simulink library "mylib"  (R2020a)
settings: Solver=VariableStepAuto  StartTime=0.0  StopTime=10.0  RelTol=1e-3
undefined symbols (not defined in the file): d_du_max_pu, dir_to_bus1, dir_to_bus_0L, dir_to_bus_2, dir_to_line1, dir_to_line_0L, dir_to_line_2, du_max_pu, du_ph_max_pu, Fi_0, Fi_T_H, Fi_T_L, Fi_T_M, I0_calc_0L, I0_comp_H, I0_comp_L, I0_comp_M, I0_max_0L, I2_max_2, I_diff1, I_diff2, I_diff3, I_diff4, I_diff5, I_diff_to, I_hight_CT1_G, I_hight_CT2_G, I_low_CT1, I_low_CT2, I_max1, I_max2, I_max3, I_max4, I_max5, I_min_sec_CT1, I_min_sec_CT2, I_unb, Iph_max_0L, Iph_max_2, jmp_in_zone, jmp_in_zone_0L, jmp_in_zone_2, K_dop, max_min1, only_K1_0L, only_K1_2, only_K2_0L, only_K2_2, only_K3_0L, only_K3_2, P_ctl_0, PQ_Fi_ctl_0, Q_ctl_0, S_set_0, set, set1, T_fast, T_I_ctl, T_off, T_on ... (+15)
libraries: $bdroot x184, powerlib_meascontrol x97
(part 4 of 14)

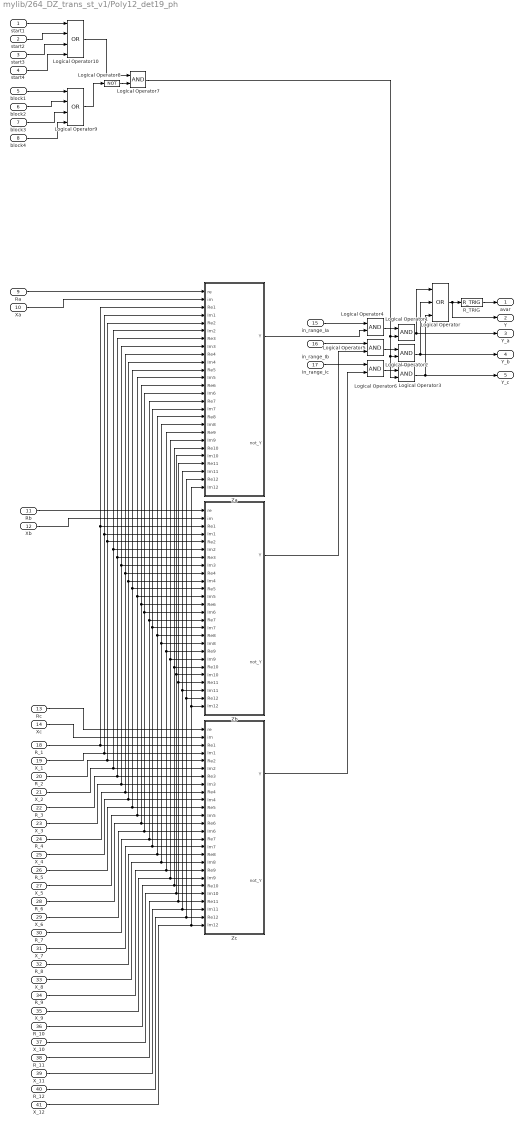
== system mylib/264_DZ_trans_st_v1/Poly12_det19_ph ==
  start1 : Inport
  start2 : Inport  Port=2
  start3 : Inport  Port=3
  start4 : Inport  Port=4
  block1 : Inport  Port=5
  block2 : Inport  Port=6
  block3 : Inport  Port=7
  block4 : Inport  Port=8
  Ra : Inport  Port=9
  Xa : Inport  Port=10
  Rb : Inport  Port=11
  Xb : Inport  Port=12
  Rc : Inport  Port=13
  Xc : Inport  Port=14
  in_range_Ia : Inport  Port=15
  in_range_Ib : Inport  Port=16
  in_range_Ic : Inport  Port=17
  R_1 : Inport  Port=18
  X_1 : Inport  Port=19
  R_2 : Inport  Port=20
  X_2 : Inport  Port=21
  R_3 : Inport  Port=22
  X_3 : Inport  Port=23
  R_4 : Inport  Port=24
  X_4 : Inport  Port=25
  R_5 : Inport  Port=26
  X_5 : Inport  Port=27
  R_6 : Inport  Port=28
  X_6 : Inport  Port=29
  R_7 : Inport  Port=30
  X_7 : Inport  Port=31
  R_8 : Inport  Port=32
  X_8 : Inport  Port=33
  R_9 : Inport  Port=34
  X_9 : Inport  Port=35
  R_10 : Inport  Port=36
  X_10 : Inport  Port=37
  R_11 : Inport  Port=38
  X_11 : Inport  Port=39
  R_12 : Inport  Port=40
  X_12 : Inport  Port=41
  Logical Operator : Logic  Operator=OR  Inputs=3  AllPortsSameDT=off  OutDataTypeStr=boolean
  Logical Operator{1..7} (7 alike) : Logic  AllPortsSameDT=off  OutDataTypeStr=boolean
  Logical Operator10 : Logic  Operator=OR  Inputs=4  AllPortsSameDT=off  OutDataTypeStr=boolean
  Logical Operator8 : Logic  Operator=NOT  AllPortsSameDT=off  OutDataTypeStr=boolean
  Logical Operator9 : Logic  Operator=OR  Inputs=4  AllPortsSameDT=off  OutDataTypeStr=boolean
  R_TRIG : $bdroot/R_TRIG  SystemSampleTime=-1  Latency=0  AutoFrameSizeCalculation=off
  Za : Subsystem
  Zb : Subsystem
  Zc : Subsystem
  avar : Outport
  Y : Outport  Port=2
  Y_a : Outport  Port=3
  Y_b : Outport  Port=4
  Y_c : Outport  Port=5
  wires:
  R_TRIG/1 -> avar/1
  Logical Operator/1 -> Y/1, R_TRIG/1
  Logical Operator1/1 -> Logical Operator/1, Y_a/1
  Logical Operator2/1 -> Logical Operator/2, Y_b/1
  Logical Operator3/1 -> Logical Operator/3, Y_c/1
  Logical Operator6/1 -> Logical Operator3/1
  Logical Operator5/1 -> Logical Operator2/1
  Logical Operator4/1 -> Logical Operator1/1
  in_range_Ia/1 -> Logical Operator4/1
  in_range_Ib/1 -> Logical Operator5/1
  in_range_Ic/1 -> Logical Operator6/1
  Logical Operator8/1 -> Logical Operator7/2
  Logical Operator7/1 -> Logical Operator3/2, Logical Operator2/2, Logical Operator1/2
  Logical Operator9/1 -> Logical Operator8/1
  Logical Operator10/1 -> Logical Operator7/1
  block1/1 -> Logical Operator9/1
  block2/1 -> Logical Operator9/2
  block3/1 -> Logical Operator9/3
  block4/1 -> Logical Operator9/4
  start4/1 -> Logical Operator10/4
  start3/1 -> Logical Operator10/3
  start2/1 -> Logical Operator10/2
  start1/1 -> Logical Operator10/1
  R_1/1 -> Za/3(Re1), Zb/3(Re1), Zc/3(Re1)
  X_1/1 -> Za/4(Im1), Zb/4(Im1), Zc/4(Im1)
  R_2/1 -> Za/5(Re2), Zb/5(Re2), Zc/5(Re2)
  X_2/1 -> Za/6(Im2), Zb/6(Im2), Zc/6(Im2)
  R_3/1 -> Za/7(Re3), Zb/7(Re3), Zc/7(Re3)
  X_3/1 -> Za/8(Im3), Zb/8(Im3), Zc/8(Im3)
  R_4/1 -> Za/9(Re4), Zb/9(Re4), Zc/9(Re4)
  X_4/1 -> Za/10(Im4), Zb/10(Im4), Zc/10(Im4)
  R_5/1 -> Za/11(Re5), Zb/11(Re5), Zc/11(Re5)
  X_5/1 -> Za/12(Im5), Zb/12(Im5), Zc/12(Im5)
  R_6/1 -> Za/13(Re6), Zb/13(Re6), Zc/13(Re6)
  X_6/1 -> Za/14(Im6), Zb/14(Im6), Zc/14(Im6)
  R_7/1 -> Za/15(Re7), Zb/15(Re7), Zc/15(Re7)
  X_7/1 -> Za/16(Im7), Zb/16(Im7), Zc/16(Im7)
  R_8/1 -> Za/17(Re8), Zb/17(Re8), Zc/17(Re8)
  X_8/1 -> Za/18(Im8), Zb/18(Im8), Zc/18(Im8)
  R_9/1 -> Za/19(Re9), Zb/19(Re9), Zc/19(Re9)
  X_9/1 -> Za/20(Im9), Zb/20(Im9), Zc/20(Im9)
  R_10/1 -> Za/21(Re10), Zb/21(Re10), Zc/21(Re10)
  X_10/1 -> Za/22(Im10), Zb/22(Im10), Zc/22(Im10)
  R_11/1 -> Za/23(Re11), Zb/23(Re11), Zc/23(Re11)
  X_11/1 -> Za/24(Im11), Zb/24(Im11), Zc/24(Im11)
  R_12/1 -> Za/25(Re12), Zb/25(Re12), Zc/25(Re12)
  X_12/1 -> Za/26(Im12), Zb/26(Im12), Zc/26(Im12)
  Xc/1 -> Zc/2(im)
  Rc/1 -> Zc/1(re)
  Rb/1 -> Zb/1(re)
  Xb/1 -> Zb/2(im)
  Xa/1 -> Za/2(im)
  Ra/1 -> Za/1(re)
  Za/1(Y) -> Logical Operator4/2
  Zb/1(Y) -> Logical Operator5/2
  Zc/1(Y) -> Logical Operator6/2

== system mylib/264_DZ_trans_st_v1/St1 ==
  fast1_time : Inport
  fast2_time : Inport  Port=2
  fast1_zero : Inport  Port=3
  fast2_zero : Inport  Port=4
  block1 : Inport  Port=5
  block2 : Inport  Port=6
  block3 : Inport  Port=7
  block4 : Inport  Port=8
  in_a : Inport  Port=9
  in_b : Inport  Port=10
  in_c : Inport  Port=11
  alt_in_a : Inport  Port=12
  alt_in_b : Inport  Port=13
  alt_in_c : Inport  Port=14
  jmp_a : Inport  Port=15
  jmp_b : Inport  Port=16
  jmp_c : Inport  Port=17
  1 : Logic  Operator=OR  Inputs=4  AllPortsSameDT=off  OutDataTypeStr=boolean
  Constant1 : Constant  Value=only_K2
  Constant2 : Constant  Value=only_K3
  Constant3 : Constant  Value=only_K1
  Constant4 : Constant  Value=jmp_in_zone
  Logical Operator1 : Logic  Operator=OR  Inputs=3  AllPortsSameDT=off  OutDataTypeStr=boolean
  Logical Operator10 : Logic  Inputs=3  AllPortsSameDT=off  OutDataTypeStr=boolean
  Logical Operator{2,4,6,11..13} (6 alike) : Logic  AllPortsSameDT=off  OutDataTypeStr=boolean
  Logical Operator{14,16..17,27..28} (5 alike) : Logic  Operator=OR  AllPortsSameDT=off  OutDataTypeStr=boolean
  Logical Operator26 : Logic  Operator=OR  Inputs=3  AllPortsSameDT=off  OutDataTypeStr=boolean
  Logical Operator3 : Logic  Operator=NOT  AllPortsSameDT=off  OutDataTypeStr=boolean
  Logical Operator5 : Logic  Operator=NOT  AllPortsSameDT=off  OutDataTypeStr=boolean
  Logical Operator7 : Logic  Operator=NOT  AllPortsSameDT=off  OutDataTypeStr=boolean
  Logical Operator8 : Logic  Inputs=3  AllPortsSameDT=off  OutDataTypeStr=boolean
  Logical Operator9 : Logic  Inputs=3  AllPortsSameDT=off  OutDataTypeStr=boolean
  R_TRIG : $bdroot/R_TRIG  SystemSampleTime=-1  Latency=0  AutoFrameSizeCalculation=off
  Subsystem : Subsystem  mask{time=[T_fast, T_st]}
      mask prompts: time "time [T_fast, T_st]"
  in_1 : Subsystem  mask{in_jmp=[T_reset]}
      mask prompts: in_jmp "in_jmp[T_reset]"
  in_2 : Subsystem  mask{in_jmp=[T_reset]}
      mask prompts: in_jmp "in_jmp[T_reset]"
  in_3 : Subsystem  mask{in_jmp=[T_reset]}
      mask prompts: in_jmp "in_jmp[T_reset]"
  k_type : Subsystem
  out_a : $bdroot/out3  out=[T_out]
  out_b : $bdroot/out3  out=[T_out]
  out_c : $bdroot/out3  out=[T_out]
  avar : Outport
  Y : Outport  Port=2
  Y_a : Outport  Port=3
  Y_b : Outport  Port=4
  Y_c : Outport  Port=5
  fast : Outport  Port=6
  fast_a : Outport  Port=7
  fast_b : Outport  Port=8
  fast_c : Outport  Port=9
  wires:
  fast1_time/1 -> Logical Operator27/1
  fast2_zero/1 -> Logical Operator28/2
  fast1_zero/1 -> Logical Operator28/1
  fast2_time/1 -> Logical Operator27/2
  block1/1 -> 1/1
  block2/1 -> 1/2
  block3/1 -> 1/3
  block4/1 -> 1/4
  in_a/1 -> in_1/2(in), Logical Operator8/1
  in_c/1 -> in_3/2(in), Logical Operator10/1
  Logical Operator26/1 -> Y/1, R_TRIG/1
  R_TRIG/1 -> avar/1
  in_b/1 -> in_2/2(in), Logical Operator9/1
  Constant4/1 -> in_3/1(jmp_in_zone), in_2/1(jmp_in_zone), in_1/1(jmp_in_zone)
  jmp_a/1 -> in_1/3(jmp)
  jmp_b/1 -> in_2/3(jmp)
  jmp_c/1 -> in_3/3(jmp)
  Logical Operator3/1 -> Logical Operator2/1
  in_1/1(Y) -> Logical Operator2/2  "Ya"
  Logical Operator5/1 -> Logical Operator4/1
  in_2/1(Y) -> Logical Operator4/2  "Yb"
  Logical Operator7/1 -> Logical Operator6/1
  in_3/1(Y) -> Logical Operator6/2  "Yc"
  1/1 -> Logical Operator7/1, Logical Operator5/1, Logical Operator3/1
  out_a/1 -> Logical Operator26/1, Y_a/1  "Y_c"
  out_b/1 -> Logical Operator26/2, Y_b/1  "Y_c"
  out_c/1 -> Logical Operator26/3, Y_c/1  "Y_c"
  Logical Operator8/1 -> out_a/1
  Logical Operator9/1 -> out_b/1
  Logical Operator10/1 -> out_c/1
  Subsystem/3(Out3) -> Logical Operator10/2
  Subsystem/2(Out2) -> Logical Operator9/2
  Subsystem/1(Out1) -> Logical Operator8/2
  Logical Operator2/1 -> Logical Operator1/1, fast_a/1, Logical Operator11/2, k_type/1(In_a)
  Logical Operator4/1 -> Logical Operator1/2, fast_b/1, Logical Operator12/2, k_type/2(In_b)
  Logical Operator6/1 -> Logical Operator1/3, fast_c/1, Logical Operator13/2, k_type/3(In_ c)
  Constant3/1 -> k_type/4(only_K1)
  Constant1/1 -> k_type/5(only_K2)
  Constant2/1 -> k_type/6(only_K3)
  k_type/1(out) -> Logical Operator10/3, Logical Operator9/3, Logical Operator8/3, Logical Operator12/1, Logical Operator13/1, Logical Operator11/1
  Logical Operator11/1 -> Logical Operator14/1
  Logical Operator12/1 -> Logical Operator16/1
  Logical Operator13/1 -> Logical Operator17/1
  Logical Operator17/1 -> Subsystem/5("In3 ")
  Logical Operator16/1 -> Subsystem/4("In2 ")
  Logical Operator14/1 -> Subsystem/3("In1 ")
  alt_in_a/1 -> Logical Operator14/2
  alt_in_b/1 -> Logical Operator16/2
  alt_in_c/1 -> Logical Operator17/2
  Logical Operator27/1 -> Subsystem/1(T_fast_time)
  Logical Operator28/1 -> Subsystem/2(T_fast_zero)
  Logical Operator1/1 -> fast/1

== system mylib/264_DZ_trans_st_v1/St2 ==
  fast1_time : Inport
  fast2_time : Inport  Port=2
  fast1_zero : Inport  Port=3
  fast2_zero : Inport  Port=4
  block1 : Inport  Port=5
  block2 : Inport  Port=6
  block3 : Inport  Port=7
  block4 : Inport  Port=8
  in_a : Inport  Port=9
  in_b : Inport  Port=10
  in_c : Inport  Port=11
  alt_in_a : Inport  Port=12
  alt_in_b : Inport  Port=13
  alt_in_c : Inport  Port=14
  jmp_a : Inport  Port=15
  jmp_b : Inport  Port=16
  jmp_c : Inport  Port=17
  1 : Logic  Operator=OR  Inputs=4  AllPortsSameDT=off  OutDataTypeStr=boolean
  Constant1 : Constant  Value=only_K2
  Constant2 : Constant  Value=only_K3
  Constant3 : Constant  Value=only_K1
  Constant4 : Constant  Value=jmp_in_zone
  Logical Operator1 : Logic  Operator=OR  Inputs=3  AllPortsSameDT=off  OutDataTypeStr=boolean
  Logical Operator10 : Logic  Inputs=3  AllPortsSameDT=off  OutDataTypeStr=boolean
  Logical Operator{2,4,6,11..13} (6 alike) : Logic  AllPortsSameDT=off  OutDataTypeStr=boolean
  Logical Operator{14,16..17,27..28} (5 alike) : Logic  Operator=OR  AllPortsSameDT=off  OutDataTypeStr=boolean
  Logical Operator26 : Logic  Operator=OR  Inputs=3  AllPortsSameDT=off  OutDataTypeStr=boolean
  Logical Operator3 : Logic  Operator=NOT  AllPortsSameDT=off  OutDataTypeStr=boolean
  Logical Operator5 : Logic  Operator=NOT  AllPortsSameDT=off  OutDataTypeStr=boolean
  Logical Operator7 : Logic  Operator=NOT  AllPortsSameDT=off  OutDataTypeStr=boolean
  Logical Operator8 : Logic  Inputs=3  AllPortsSameDT=off  OutDataTypeStr=boolean
  Logical Operator9 : Logic  Inputs=3  AllPortsSameDT=off  OutDataTypeStr=boolean
  R_TRIG : $bdroot/R_TRIG  SystemSampleTime=-1  Latency=0  AutoFrameSizeCalculation=off
  Subsystem : Subsystem  mask{time=[T_fast, T_st]}
      mask prompts: time "time [T_fast, T_st]"
  in_1 : Subsystem  mask{in_jmp=[T_reset]}
      mask prompts: in_jmp "in_jmp[T_reset]"
  in_2 : Subsystem  mask{in_jmp=[T_reset]}
      mask prompts: in_jmp "in_jmp[T_reset]"
  in_3 : Subsystem  mask{in_jmp=[T_reset]}
      mask prompts: in_jmp "in_jmp[T_reset]"
  k_type : Subsystem
  out_a : $bdroot/out3  out=[T_out]
  out_b : $bdroot/out3  out=[T_out]
  out_c : $bdroot/out3  out=[T_out]
  avar : Outport
  Y : Outport  Port=2
  Y_a : Outport  Port=3
  Y_b : Outport  Port=4
  Y_c : Outport  Port=5
  fast : Outport  Port=6
  fast_a : Outport  Port=7
  fast_b : Outport  Port=8
  fast_c : Outport  Port=9
  wires:
  fast1_time/1 -> Logical Operator27/1
  fast2_zero/1 -> Logical Operator28/2
  fast1_zero/1 -> Logical Operator28/1
  fast2_time/1 -> Logical Operator27/2
  block1/1 -> 1/1
  block2/1 -> 1/2
  block3/1 -> 1/3
  block4/1 -> 1/4
  in_a/1 -> in_1/2(in), Logical Operator8/1
  in_c/1 -> in_3/2(in), Logical Operator10/1
  Logical Operator26/1 -> Y/1, R_TRIG/1
  R_TRIG/1 -> avar/1
  in_b/1 -> in_2/2(in), Logical Operator9/1
  Constant4/1 -> in_3/1(jmp_in_zone), in_2/1(jmp_in_zone), in_1/1(jmp_in_zone)
  jmp_a/1 -> in_1/3(jmp)
  jmp_b/1 -> in_2/3(jmp)
  jmp_c/1 -> in_3/3(jmp)
  Logical Operator3/1 -> Logical Operator2/1
  in_1/1(Y) -> Logical Operator2/2  "Ya"
  Logical Operator5/1 -> Logical Operator4/1
  in_2/1(Y) -> Logical Operator4/2  "Yb"
  Logical Operator7/1 -> Logical Operator6/1
  in_3/1(Y) -> Logical Operator6/2  "Yc"
  1/1 -> Logical Operator7/1, Logical Operator5/1, Logical Operator3/1
  out_a/1 -> Logical Operator26/1, Y_a/1  "Y_c"
  out_b/1 -> Logical Operator26/2, Y_b/1  "Y_c"
  out_c/1 -> Logical Operator26/3, Y_c/1  "Y_c"
  Logical Operator8/1 -> out_a/1
  Logical Operator9/1 -> out_b/1
  Logical Operator10/1 -> out_c/1
  Subsystem/3(Out3) -> Logical Operator10/2
  Subsystem/2(Out2) -> Logical Operator9/2
  Subsystem/1(Out1) -> Logical Operator8/2
  Logical Operator2/1 -> Logical Operator1/1, fast_a/1, Logical Operator11/2, k_type/1(In_a)
  Logical Operator4/1 -> Logical Operator1/2, fast_b/1, Logical Operator12/2, k_type/2(In_b)
  Logical Operator6/1 -> Logical Operator1/3, fast_c/1, Logical Operator13/2, k_type/3(In_ c)
  Constant3/1 -> k_type/4(only_K1)
  Constant1/1 -> k_type/5(only_K2)
  Constant2/1 -> k_type/6(only_K3)
  k_type/1(out) -> Logical Operator10/3, Logical Operator9/3, Logical Operator8/3, Logical Operator12/1, Logical Operator13/1, Logical Operator11/1
  Logical Operator11/1 -> Logical Operator14/1
  Logical Operator12/1 -> Logical Operator16/1
  Logical Operator13/1 -> Logical Operator17/1
  Logical Operator17/1 -> Subsystem/5("In3 ")
  Logical Operator16/1 -> Subsystem/4("In2 ")
  Logical Operator14/1 -> Subsystem/3("In1 ")
  alt_in_a/1 -> Logical Operator14/2
  alt_in_b/1 -> Logical Operator16/2
  alt_in_c/1 -> Logical Operator17/2
  Logical Operator27/1 -> Subsystem/1(T_fast_time)
  Logical Operator28/1 -> Subsystem/2(T_fast_zero)
  Logical Operator1/1 -> fast/1

== system mylib/264_DZ_trans_st_v1/St3 ==
  fast1_time : Inport
  fast2_time : Inport  Port=2
  fast1_zero : Inport  Port=3
  fast2_zero : Inport  Port=4
  block1 : Inport  Port=5
  block2 : Inport  Port=6
  block3 : Inport  Port=7
  block4 : Inport  Port=8
  in_a : Inport  Port=9
  in_b : Inport  Port=10
  in_c : Inport  Port=11
  alt_in_a : Inport  Port=12
  alt_in_b : Inport  Port=13
  alt_in_c : Inport  Port=14
  jmp_a : Inport  Port=15
  jmp_b : Inport  Port=16
  jmp_c : Inport  Port=17
  1 : Logic  Operator=OR  Inputs=4  AllPortsSameDT=off  OutDataTypeStr=boolean
  Constant1 : Constant  Value=only_K2
  Constant2 : Constant  Value=only_K3
  Constant3 : Constant  Value=only_K1
  Constant4 : Constant  Value=jmp_in_zone
  Logical Operator1 : Logic  Operator=OR  Inputs=3  AllPortsSameDT=off  OutDataTypeStr=boolean
  Logical Operator10 : Logic  Inputs=3  AllPortsSameDT=off  OutDataTypeStr=boolean
  Logical Operator{2,4,6,11..13} (6 alike) : Logic  AllPortsSameDT=off  OutDataTypeStr=boolean
  Logical Operator{14,16..17,27..28} (5 alike) : Logic  Operator=OR  AllPortsSameDT=off  OutDataTypeStr=boolean
  Logical Operator26 : Logic  Operator=OR  Inputs=3  AllPortsSameDT=off  OutDataTypeStr=boolean
  Logical Operator3 : Logic  Operator=NOT  AllPortsSameDT=off  OutDataTypeStr=boolean
  Logical Operator5 : Logic  Operator=NOT  AllPortsSameDT=off  OutDataTypeStr=boolean
  Logical Operator7 : Logic  Operator=NOT  AllPortsSameDT=off  OutDataTypeStr=boolean
  Logical Operator8 : Logic  Inputs=3  AllPortsSameDT=off  OutDataTypeStr=boolean
  Logical Operator9 : Logic  Inputs=3  AllPortsSameDT=off  OutDataTypeStr=boolean
  R_TRIG : $bdroot/R_TRIG  SystemSampleTime=-1  Latency=0  AutoFrameSizeCalculation=off
  Subsystem : Subsystem  mask{time=[T_fast, T_st]}
      mask prompts: time "time [T_fast, T_st]"
  in_1 : Subsystem  mask{in_jmp=[T_reset]}
      mask prompts: in_jmp "in_jmp[T_reset]"
  in_2 : Subsystem  mask{in_jmp=[T_reset]}
      mask prompts: in_jmp "in_jmp[T_reset]"
  in_3 : Subsystem  mask{in_jmp=[T_reset]}
      mask prompts: in_jmp "in_jmp[T_reset]"
  k_type : Subsystem
  out_a : $bdroot/out3  out=[T_out]
  out_b : $bdroot/out3  out=[T_out]
  out_c : $bdroot/out3  out=[T_out]
  avar : Outport
  Y : Outport  Port=2
  Y_a : Outport  Port=3
  Y_b : Outport  Port=4
  Y_c : Outport  Port=5
  fast : Outport  Port=6
  fast_a : Outport  Port=7
  fast_b : Outport  Port=8
  fast_c : Outport  Port=9
  wires:
  fast1_time/1 -> Logical Operator27/1
  fast2_zero/1 -> Logical Operator28/2
  fast1_zero/1 -> Logical Operator28/1
  fast2_time/1 -> Logical Operator27/2
  block1/1 -> 1/1
  block2/1 -> 1/2
  block3/1 -> 1/3
  block4/1 -> 1/4
  in_a/1 -> in_1/2(in), Logical Operator8/1
  in_c/1 -> in_3/2(in), Logical Operator10/1
  Logical Operator26/1 -> Y/1, R_TRIG/1
  R_TRIG/1 -> avar/1
  in_b/1 -> in_2/2(in), Logical Operator9/1
  Constant4/1 -> in_3/1(jmp_in_zone), in_2/1(jmp_in_zone), in_1/1(jmp_in_zone)
  jmp_a/1 -> in_1/3(jmp)
  jmp_b/1 -> in_2/3(jmp)
  jmp_c/1 -> in_3/3(jmp)
  Logical Operator3/1 -> Logical Operator2/1
  in_1/1(Y) -> Logical Operator2/2  "Ya"
  Logical Operator5/1 -> Logical Operator4/1
  in_2/1(Y) -> Logical Operator4/2  "Yb"
  Logical Operator7/1 -> Logical Operator6/1
  in_3/1(Y) -> Logical Operator6/2  "Yc"
  1/1 -> Logical Operator7/1, Logical Operator5/1, Logical Operator3/1
  out_a/1 -> Logical Operator26/1, Y_a/1  "Y_c"
  out_b/1 -> Logical Operator26/2, Y_b/1  "Y_c"
  out_c/1 -> Logical Operator26/3, Y_c/1  "Y_c"
  Logical Operator8/1 -> out_a/1
  Logical Operator9/1 -> out_b/1
  Logical Operator10/1 -> out_c/1
  Subsystem/3(Out3) -> Logical Operator10/2
  Subsystem/2(Out2) -> Logical Operator9/2
  Subsystem/1(Out1) -> Logical Operator8/2
  Logical Operator2/1 -> Logical Operator1/1, fast_a/1, Logical Operator11/2, k_type/1(In_a)
  Logical Operator4/1 -> Logical Operator1/2, fast_b/1, Logical Operator12/2, k_type/2(In_b)
  Logical Operator6/1 -> Logical Operator1/3, fast_c/1, Logical Operator13/2, k_type/3(In_ c)
  Constant3/1 -> k_type/4(only_K1)
  Constant1/1 -> k_type/5(only_K2)
  Constant2/1 -> k_type/6(only_K3)
  k_type/1(out) -> Logical Operator10/3, Logical Operator9/3, Logical Operator8/3, Logical Operator12/1, Logical Operator13/1, Logical Operator11/1
  Logical Operator11/1 -> Logical Operator14/1
  Logical Operator12/1 -> Logical Operator16/1
  Logical Operator13/1 -> Logical Operator17/1
  Logical Operator17/1 -> Subsystem/5("In3 ")
  Logical Operator16/1 -> Subsystem/4("In2 ")
  Logical Operator14/1 -> Subsystem/3("In1 ")
  alt_in_a/1 -> Logical Operator14/2
  alt_in_b/1 -> Logical Operator16/2
  alt_in_c/1 -> Logical Operator17/2
  Logical Operator27/1 -> Subsystem/1(T_fast_time)
  Logical Operator28/1 -> Subsystem/2(T_fast_zero)
  Logical Operator1/1 -> fast/1

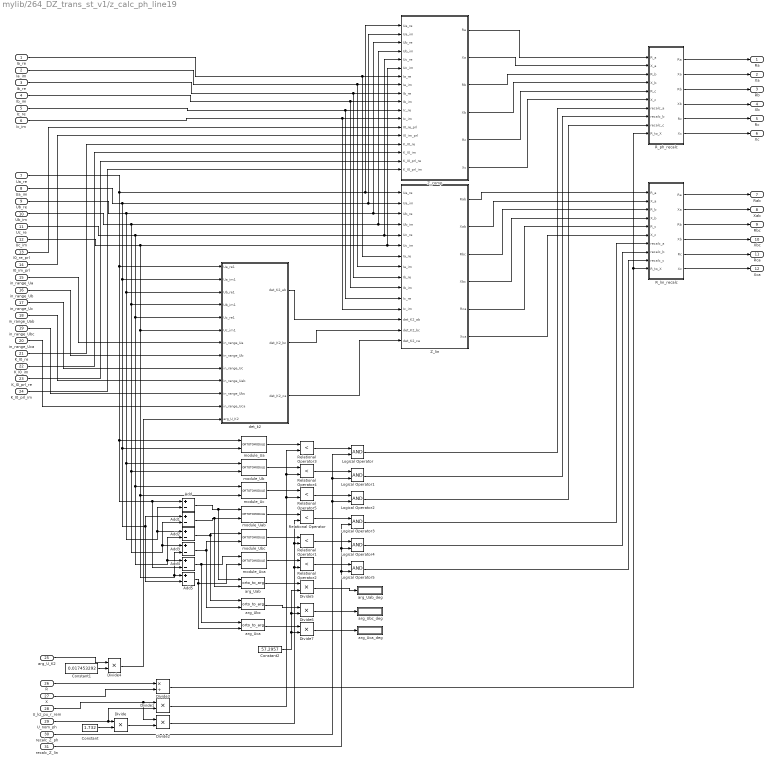
== system mylib/264_DZ_trans_st_v1/z_calc_ph_line19 ==
  Ia_re : Inport
  Ia_im : Inport  Port=2
  Ib_re : Inport  Port=3
  Ib_im : Inport  Port=4
  Ic_re : Inport  Port=5
  Ic_im : Inport  Port=6
  Ua_re : Inport  Port=7
  Ua_im : Inport  Port=8
  Ub_re : Inport  Port=9
  Ub_im : Inport  Port=10
  Uc_re : Inport  Port=11
  Uc_im : Inport  Port=12
  I0_re_prl : Inport  Port=13
  I0_im_prl : Inport  Port=14
  in_range_Ua : Inport  Port=15
  in_range_Ub : Inport  Port=16
  in_range_Uc : Inport  Port=17
  in_range_Uab : Inport  Port=18
  in_range_Ubc : Inport  Port=19
  in_range_Uca : Inport  Port=20
  K_I0_re : Inport  Port=21
  K_I0_im : Inport  Port=22
  K_I0_prl_re : Inport  Port=23
  K_I0_prl_im : Inport  Port=24
  arg_U_K2 : Inport  Port=25
  R : Inport  Port=26
  X : Inport  Port=27
  U_kz_pu_r_rem : Inport  Port=28
  U_nom_ph : Inport  Port=29
  recalc_Z_ph : Inport  Port=30
  recalc_Z_lin : Inport  Port=31
  Add{,1..5} (6 alike) : Sum  Inputs=+-
  Constant : Constant  Value=1.732
  Constant1 : Constant  Value=0.017453292
  Constant2 : Constant  Value=57.2957
  Divide{,1..2,4..7} (7 alike) : Product  Inputs=**
  Divide3 : Product  Inputs=*/
  Logical Operator{,1..5} (6 alike) : Logic  AllPortsSameDT=off  OutDataTypeStr=boolean
  R_lin_recalc : Subsystem
  R_ph_recalc : Subsystem
  Relational Operator{,1..5} (6 alike) : RelationalOperator  Operator=<  OutDataTypeStr=boolean  RndMeth=Simplest
  Z_comp : Subsystem
  Z_lin : Subsystem
  arg_Uab : $bdroot/orto_to_arg  SystemSampleTime=-1  Latency=0  AutoFrameSizeCalculation=off
  arg_Uab_deg : Display
  arg_Ubc : $bdroot/orto_to_arg  SystemSampleTime=-1  Latency=0  AutoFrameSizeCalculation=off
  arg_Ubc_deg : Display
  arg_Uca : $bdroot/orto_to_arg  SystemSampleTime=-1  Latency=0  AutoFrameSizeCalculation=off
  arg_Uca_deg : Display
  det_k2 : Subsystem
  module_Ua : $bdroot/ORTOTOMODULE  SystemSampleTime=-1  Latency=0  AutoFrameSizeCalculation=off
  module_Uab : $bdroot/ORTOTOMODULE  SystemSampleTime=-1  Latency=0  AutoFrameSizeCalculation=off
  module_Ub : $bdroot/ORTOTOMODULE  SystemSampleTime=-1  Latency=0  AutoFrameSizeCalculation=off
  module_Ubc : $bdroot/ORTOTOMODULE  SystemSampleTime=-1  Latency=0  AutoFrameSizeCalculation=off
  module_Uc : $bdroot/ORTOTOMODULE  SystemSampleTime=-1  Latency=0  AutoFrameSizeCalculation=off
  module_Uca : $bdroot/ORTOTOMODULE  SystemSampleTime=-1  Latency=0  AutoFrameSizeCalculation=off
  Ra : Outport
  Xa : Outport  Port=2
  Rb : Outport  Port=3
  Xb : Outport  Port=4
  Rc : Outport  Port=5
  Xc : Outport  Port=6
  Rab : Outport  Port=7
  Xab : Outport  Port=8
  Rbc : Outport  Port=9
  Xbc : Outport  Port=10
  Rca : Outport  Port=11
  Xca : Outport  Port=12
  wires:
  Ua_re/1 -> Z_lin/1(Ua_re), Z_comp/1(Ua_re), module_Ua/1, Add4/2, Add/1, det_k2/1(Ua_re1)
  Ub_re/1 -> det_k2/3(Ub_re1), Add/2, Add2/1, module_Ub/1, Z_comp/3(Ub_re), Z_lin/3(Ub_re)
  Ua_im/1 -> det_k2/2(Ua_im1), Add1/1, Add5/2, module_Ua/2, Z_comp/2(Ua_im), Z_lin/2(Ua_im)
  Ub_im/1 -> det_k2/4(Ub_im1), Add1/2, Add3/1, module_Ub/2, Z_comp/4(Ub_im), Z_lin/4(Ub_im)
  Uc_re/1 -> det_k2/5(Uc_re1), Add2/2, Add4/1, module_Uc/1, Z_comp/5(Uc_re), Z_lin/5(Uc_re)
  Uc_im/1 -> det_k2/6(Uc_im1), Add3/2, Add5/1, module_Uc/2, Z_comp/6(Uc_im), Z_lin/6(Uc_im)
  Add1/1 -> arg_Uab/2, module_Uab/2
  Add/1 -> module_Uab/1, arg_Uab/1
  Add2/1 -> arg_Ubc/1, module_Ubc/1
  Add3/1 -> arg_Ubc/2, module_Ubc/2
  Add4/1 -> arg_Uca/1, module_Uca/1
  Add5/1 -> arg_Uca/2, module_Uca/2
  module_Uab/1 -> Relational Operator/1
  module_Uca/1 -> Relational Operator2/1
  module_Ubc/1 -> Relational Operator1/1
  Constant/1 -> Divide/2
  U_kz_pu_r_rem/1 -> Divide2/1, Divide1/1
  U_nom_ph/1 -> Divide1/2, Divide/1
  Divide/1 -> Divide2/2
  X/1 -> Divide3/2
  R/1 -> Divide3/1
  arg_U_K2/1 -> Divide4/1
  Constant1/1 -> Divide4/2
  module_Ua/1 -> Relational Operator3/1
  module_Ub/1 -> Relational Operator4/1
  module_Uc/1 -> Relational Operator5/1
  Relational Operator3/1 -> Logical Operator/1
  Relational Operator4/1 -> Logical Operator1/1
  Relational Operator5/1 -> Logical Operator2/1
  Relational Operator/1 -> Logical Operator3/1
  Relational Operator1/1 -> Logical Operator4/1
  Relational Operator2/1 -> Logical Operator5/1
  recalc_Z_ph/1 -> Logical Operator2/2, Logical Operator1/2, Logical Operator/2
  recalc_Z_lin/1 -> Logical Operator5/2, Logical Operator4/2, Logical Operator3/2
  arg_Uab/1 -> Divide5/1
  arg_Ubc/1 -> Divide6/1
  arg_Uca/1 -> Divide7/1
  Constant2/1 -> Divide5/2, Divide6/2, Divide7/2
  Divide5/1 -> arg_Uab_deg/1
  Divide6/1 -> arg_Ubc_deg/1
  Divide7/1 -> arg_Uca_deg/1
  Divide1/1 -> Relational Operator5/2, Relational Operator3/2, Relational Operator4/2
  Divide2/1 -> Relational Operator2/2, Relational Operator1/2, Relational Operator/2
  R_ph_recalc/1(Ra) -> Ra/1
  R_ph_recalc/6(Xc) -> Xc/1
  R_ph_recalc/5(Rc) -> Rc/1
  R_ph_recalc/4(Xb) -> Xb/1
  R_ph_recalc/3(Rb) -> Rb/1
  R_ph_recalc/2(Xa) -> Xa/1
  R_lin_recalc/1(Ra) -> Rab/1
  R_lin_recalc/6(Xc) -> Xca/1
  R_lin_recalc/5(Rc) -> Rca/1
  R_lin_recalc/4(Xb) -> Xbc/1
  R_lin_recalc/3(Rb) -> Rbc/1
  R_lin_recalc/2(Xa) -> Xab/1
  Z_lin/1(Rab) -> R_lin_recalc/1(R_a)
  Z_lin/2(Xab) -> R_lin_recalc/2(X_a)
  Z_lin/3(Rbc) -> R_lin_recalc/3(R_b)
  Z_lin/4(Xbc) -> R_lin_recalc/4(X_b)
  Z_lin/5(Rca) -> R_lin_recalc/5(R_c)
  Z_lin/6(Xca) -> R_lin_recalc/6(X_c)
  Z_comp/1(Ra) -> R_ph_recalc/1(R_a)
  Z_comp/2(Xa) -> R_ph_recalc/2(X_a)
  Z_comp/3(Rb) -> R_ph_recalc/3(R_b)
  Z_comp/4(Xb) -> R_ph_recalc/4(X_b)
  Z_comp/5(Rc) -> R_ph_recalc/5(R_c)
  Z_comp/6(Xc) -> R_ph_recalc/6(X_c)
  det_k2/1(det_K2_ab) -> Z_lin/13(det_K2_ab)
  det_k2/2(det_K2_bc) -> Z_lin/14(det_K2_bc)
  det_k2/3(det_K2_ca) -> Z_lin/15(det_K2_ca)
  Ia_re/1 -> Z_lin/7(Ia_re), Z_comp/7(Ia_re)
  Ia_im/1 -> Z_lin/8(Ia_im), Z_comp/8(Ia_im)
  Ib_re/1 -> Z_lin/9(Ib_re), Z_comp/9(Ib_re)
  Ib_im/1 -> Z_lin/10(Ib_im), Z_comp/10(Ib_im)
  Ic_re/1 -> Z_lin/11(Ic_re), Z_comp/11(Ic_re)
  Ic_im/1 -> Z_lin/12(Ic_im), Z_comp/12(Ic_im)
  I0_re_prl/1 -> Z_comp/13(I0_re_prl)
  I0_im_prl/1 -> Z_comp/14(I0_im_prl)
  in_range_Ua/1 -> det_k2/7(in_range_Ua)
  in_range_Ub/1 -> det_k2/8(in_range_Ub)
  in_range_Uc/1 -> det_k2/9(in_range_Uc)
  in_range_Uab/1 -> det_k2/10(in_range_Uab)
  in_range_Ubc/1 -> det_k2/11(in_range_Ubc)
  in_range_Uca/1 -> det_k2/12(in_range_Uca)
  K_I0_re/1 -> Z_comp/15(K_I0_re)
  K_I0_im/1 -> Z_comp/16(K_I0_im)
  K_I0_prl_re/1 -> Z_comp/17(K_I0_prl_re)
  K_I0_prl_im/1 -> Z_comp/18(K_I0_prl_im)
  Divide4/1 -> det_k2/13(arg_U_K2)
  Divide3/1 -> R_ph_recalc/10(R_to_X), R_lin_recalc/10(R_to_X)
  Logical Operator/1 -> R_ph_recalc/7(recalc_a)
  Logical Operator1/1 -> R_ph_recalc/8(recalc_b)
  Logical Operator2/1 -> R_ph_recalc/9(recalc_c)
  Logical Operator3/1 -> R_lin_recalc/7(recalc_a)
  Logical Operator4/1 -> R_lin_recalc/8(recalc_b)
  Logical Operator5/1 -> R_lin_recalc/9(recalc_c)

== system mylib/278_dzt_v1/K_T_HL ==
  hight : Inport
  low : Inport  Port=2
  1 : Switch  Criteria=u2 > Threshold
  15 : RelationalOperator  Operator===  OutDataTypeStr=boolean  RndMeth=Nearest
  16 : Product  Inputs=*/  RndMeth=Zero  SaturateOnIntegerOverflow=on
  17 : RelationalOperator  Operator===  OutDataTypeStr=boolean  RndMeth=Nearest
  18 : Logic  Operator=OR  AllPortsSameDT=off  OutDataTypeStr=boolean
  19 : Constant
  20 : Constant  Value=0
  K : Outport
  wires:
  hight/1 -> 15/1, 16/1
  18/1 -> 1/2
  20/1 -> 17/2, 15/2
  16/1 -> 1/3
  17/1 -> 18/2
  19/1 -> 1/1
  15/1 -> 18/1
  low/1 -> 17/1, 16/2
  1/1 -> K/1

== system mylib/278_dzt_v1/K_T_HM ==
  hight : Inport
  low : Inport  Port=2
  1 : Switch  Criteria=u2 > Threshold
  15 : RelationalOperator  Operator===  OutDataTypeStr=boolean  RndMeth=Nearest
  16 : Product  Inputs=*/  RndMeth=Zero  SaturateOnIntegerOverflow=on
  17 : RelationalOperator  Operator===  OutDataTypeStr=boolean  RndMeth=Nearest
  18 : Logic  Operator=OR  AllPortsSameDT=off  OutDataTypeStr=boolean
  19 : Constant
  20 : Constant  Value=0
  K : Outport
  wires:
  hight/1 -> 15/1, 16/1
  18/1 -> 1/2
  20/1 -> 17/2, 15/2
  16/1 -> 1/3
  17/1 -> 18/2
  19/1 -> 1/1
  15/1 -> 18/1
  low/1 -> 17/1, 16/2
  1/1 -> K/1

== system mylib/278_dzt_v1/diff_brake ==
  Ia_max : Inport
  Ib_max : Inport  Port=2
  Ic_max : Inport  Port=3
  I_diff_to : Inport  Port=4
  I_diff_1 : Inport  Port=5
  I_max_1 : Inport  Port=6
  I_diff_2 : Inport  Port=7
  I_max_2 : Inport  Port=8
  I_diff_3 : Inport  Port=9
  I_max_3 : Inport  Port=10
  I_diff_4 : Inport  Port=11
  I_max_4 : Inport  Port=12
  I_diff_5 : Inport  Port=13
  I_max_5 : Inport  Port=14
  calc_brake_Ia : Subsystem
  calc_brake_Ib : Subsystem
  calc_brake_Ic : Subsystem
  Ia_brake : Outport
  Ib_brake : Outport  Port=2
  Ic_brake : Outport  Port=3
  wires:
  calc_brake_Ib/1(I_brake) -> Ib_brake/1
  Ib_max/1 -> calc_brake_Ib/1(I_max)
  I_diff_2/1 -> calc_brake_Ic/5(I_diff_2), calc_brake_Ia/5(I_diff_2), calc_brake_Ib/5(I_diff_2)
  I_max_1/1 -> calc_brake_Ic/4(I_max_1), calc_brake_Ib/4(I_max_1), calc_brake_Ia/4(I_max_1)
  I_max_2/1 -> calc_brake_Ic/6(I_max_2), calc_brake_Ib/6(I_max_2), calc_brake_Ia/6(I_max_2)
  I_diff_3/1 -> calc_brake_Ic/7(I_diff_3), calc_brake_Ib/7(I_diff_3), calc_brake_Ia/7(I_diff_3)
  I_max_3/1 -> calc_brake_Ic/8(I_max_3), calc_brake_Ib/8(I_max_3), calc_brake_Ia/8(I_max_3)
  I_diff_4/1 -> calc_brake_Ic/9(I_diff_4), calc_brake_Ib/9(I_diff_4), calc_brake_Ia/9(I_diff_4)
  I_max_4/1 -> calc_brake_Ic/10(I_max_4), calc_brake_Ib/10(I_max_4), calc_brake_Ia/10(I_max_4)
  I_diff_5/1 -> calc_brake_Ic/11(I_diff_5), calc_brake_Ib/11(I_diff_5), calc_brake_Ia/11(I_diff_5)
  I_max_5/1 -> calc_brake_Ic/12(I_max_5), calc_brake_Ib/12(I_max_5), calc_brake_Ia/12(I_max_5)
  I_diff_1/1 -> calc_brake_Ic/3(I_diff_1), calc_brake_Ib/3(I_diff_1), calc_brake_Ia/3(I_diff_1)
  I_diff_to/1 -> calc_brake_Ib/2(I_diff_to), calc_brake_Ia/2(I_diff_to), calc_brake_Ic/2(I_diff_to)
  Ic_max/1 -> calc_brake_Ic/1(I_max)
  Ia_max/1 -> calc_brake_Ia/1(I_max)
  calc_brake_Ia/1(I_brake) -> Ia_brake/1
  calc_brake_Ic/1(I_brake) -> Ic_brake/1

== system mylib/278_dzt_v1/diff_comp18_ph ==
  Ia_diff : Inport
  Ib_diff : Inport  Port=2
  Ic_diff : Inport  Port=3
  Ia_brake : Inport  Port=4
  Ib_brake : Inport  Port=5
  Ic_brake : Inport  Port=6
  I_diff_to : Inport  Port=7
  diff_comp_a : Subsystem
  diff_comp_b : Subsystem
  diff_comp_c : Subsystem
  Y_a : Outport
  Y_b : Outport  Port=2
  Y_c : Outport  Port=3
  wires:
  I_diff_to/1 -> diff_comp_b/3(I_diff_to), diff_comp_a/3(I_diff_to), diff_comp_c/3(I_diff_to)
  Ic_brake/1 -> diff_comp_c/2(I_brake)
  Ib_brake/1 -> diff_comp_b/2(I_brake)
  Ia_brake/1 -> diff_comp_a/2(I_brake)
  Ic_diff/1 -> diff_comp_c/1(I_diff)
  Ib_diff/1 -> diff_comp_b/1(I_diff)
  Ia_diff/1 -> diff_comp_a/1(I_diff)
  diff_comp_a/1(Y) -> Y_a/1
  diff_comp_b/1(Y) -> Y_b/1
  diff_comp_c/1(Y) -> Y_c/1

== system mylib/278_dzt_v1/diff_trans_calc_H ==
  Ia_re_diff_in : Inport
  Ia_im_diff_in : Inport  Port=2
  Ia_re_max_in : Inport  Port=3
  Ia_im_max_in : Inport  Port=4
  Ib_re_diff_in : Inport  Port=5
  Ib_im_diff_in : Inport  Port=6
  Ib_re_max_in : Inport  Port=7
  Ib_im_max_in : Inport  Port=8
  Ic_re_diff_in : Inport  Port=9
  Ic_im_diff_in : Inport  Port=10
  Ic_re_max_in : Inport  Port=11
  Ic_im_max_in : Inport  Port=12
  Ia_zero_in : Inport  Port=13
  Ib_zero_in : Inport  Port=14
  Ic_zero_in : Inport  Port=15
  I_all_zero_in : Inport  Port=16
  Ia_re : Inport  Port=17
  Ia_im : Inport  Port=18
  Ib_re : Inport  Port=19
  Ib_im : Inport  Port=20
  Ic_re : Inport  Port=21
  Ic_im : Inport  Port=22
  jmp_a : Inport  Port=23
  jmp_b : Inport  Port=24
  jmp_c : Inport  Port=25
  in_range_Ia : Inport  Port=26
  in_range_Ib : Inport  Port=27
  in_range_Ic : Inport  Port=28
  K_T : Inport  Port=29
  I0_comp : Inport  Port=30
  Fi_T : Inport  Port=31
  1 : Constant  Value=0
  2 : Constant
  6 : Constant  Value=0
  9 : Constant
  Ia_calc : Subsystem
  Ia_diff_calc : Subsystem
  Ib_calc : Subsystem
  Ib_diff_calc : Subsystem
  Ic_calc : Subsystem
  Ic_diff_calc : Subsystem
  jmp_cnt18_ph : Subsystem
  simpcomp : Subsystem
  Ia_re_diff : Outport
  Ia_im_diff : Outport  Port=2
  Ia_re_max : Outport  Port=3
  Ia_im_max : Outport  Port=4
  Ib_re_diff : Outport  Port=5
  Ib_im_diff : Outport  Port=6
  Ib_re_max : Outport  Port=7
  Ib_im_max : Outport  Port=8
  Ic_re_diff : Outport  Port=9
  Ic_im_diff : Outport  Port=10
  Ic_re_max : Outport  Port=11
  Ic_im_max : Outport  Port=12
  Ia_zero : Outport  Port=13
  Ib_zero : Outport  Port=14
  Ic_zero : Outport  Port=15
  I_all_zero : Outport  Port=16
  wires:
  Ia_re/1 -> simpcomp/1(FAre), Ia_calc/1(I_re_in)
  I_all_zero_in/1 -> jmp_cnt18_ph/6(Iall_zero_in)
  Ic_zero_in/1 -> jmp_cnt18_ph/5(Ic_zero_in)
  Ib_zero_in/1 -> jmp_cnt18_ph/4(Ib_zero_in)
  Ia_zero_in/1 -> jmp_cnt18_ph/3(Ia_zero_in)
  Ic_im_max_in/1 -> Ic_diff_calc/7(I_im_max_in)
  Ic_re_max_in/1 -> Ic_diff_calc/6(I_re_max_in)
  Ic_im_diff_in/1 -> Ic_diff_calc/2(I_im_1)
  Ic_re_diff_in/1 -> Ic_diff_calc/1(I_re_1)
  Ib_im_max_in/1 -> Ib_diff_calc/7(I_im_max_in)
  Ib_re_max_in/1 -> Ib_diff_calc/6(I_re_max_in)
  Ib_im_diff_in/1 -> Ib_diff_calc/2(I_im_1)
  Ib_re_diff_in/1 -> Ib_diff_calc/1(I_re_1)
  Ia_im_max_in/1 -> Ia_diff_calc/7(I_im_max_in)
  Ia_re_max_in/1 -> Ia_diff_calc/6(I_re_max_in)
  Ia_im_diff_in/1 -> Ia_diff_calc/2(I_im_1)
  Ia_re_diff_in/1 -> Ia_diff_calc/1(I_re_1)
  2/1 -> Ia_diff_calc/5(fix), Ib_diff_calc/5(fix), jmp_cnt18_ph/13(fix), Ic_diff_calc/5(fix)
  1/1 -> jmp_cnt18_ph/2(cnt_jmp_in), jmp_cnt18_ph/1(cnt_jmp0_in)
  Ia_calc/1(I_re) -> Ia_diff_calc/3(I_re_2)
  Ia_calc/2(I_im) -> Ia_diff_calc/4(I_im_2)
  Ib_calc/1(I_re) -> Ib_diff_calc/3(I_re_2)
  Ib_calc/2(I_im) -> Ib_diff_calc/4(I_im_2)
  Ic_calc/1(I_re) -> Ic_diff_calc/3(I_re_2)
  Ic_calc/2(I_im) -> Ic_diff_calc/4(I_im_2)
  Ia_diff_calc/1(I_re_diff) -> Ia_re_diff/1
  Ia_diff_calc/2(I_im_diff1) -> Ia_im_diff/1
  Ia_diff_calc/3(I_re_max) -> Ia_re_max/1
  Ia_diff_calc/4(I_im_max) -> Ia_im_max/1
  Ib_diff_calc/4(I_im_max) -> Ib_im_max/1
  Ib_diff_calc/3(I_re_max) -> Ib_re_max/1
  Ib_diff_calc/2(I_im_diff1) -> Ib_im_diff/1
  Ib_diff_calc/1(I_re_diff) -> Ib_re_diff/1
  Ic_diff_calc/4(I_im_max) -> Ic_im_max/1
  Ic_diff_calc/3(I_re_max) -> Ic_re_max/1
  Ic_diff_calc/2(I_im_diff1) -> Ic_im_diff/1
  Ic_diff_calc/1(I_re_diff) -> Ic_re_diff/1
  jmp_cnt18_ph/6(Iall_zero) -> I_all_zero/1
  jmp_cnt18_ph/5(Ic_zero) -> Ic_zero/1
  jmp_cnt18_ph/4(Ib_zero) -> Ib_zero/1
  jmp_cnt18_ph/3(Ia_zero) -> Ia_zero/1
  Ia_im/1 -> simpcomp/2(FAim), Ia_calc/2(I_im_in)
  Ib_re/1 -> simpcomp/3(FBre), Ib_calc/1(I_re_in)
  Ib_im/1 -> simpcomp/4(FBim), Ib_calc/2(I_im_in)
  Ic_re/1 -> simpcomp/5(FCre), Ic_calc/1(I_re_in)
  Ic_im/1 -> simpcomp/6(FCim), Ic_calc/2(I_im_in)
  jmp_a/1 -> jmp_cnt18_ph/10(jmp_Ia)
  jmp_b/1 -> jmp_cnt18_ph/11(jmp_Ib)
  jmp_c/1 -> jmp_cnt18_ph/12(jmp_Ic)
  in_range_Ib/1 -> jmp_cnt18_ph/8(in_range_Ib), Ib_diff_calc/8(in_range_I)
  in_range_Ic/1 -> Ic_diff_calc/8(in_range_I), jmp_cnt18_ph/9(in_range_Ic)
  simpcomp/2(F0im) -> Ib_calc/4(I30_im), Ia_calc/4(I30_im), Ic_calc/4(I30_im)
  simpcomp/1(F0re) -> Ia_calc/3(I30_re), Ib_calc/3(I30_re), Ic_calc/3(I30_re)
  in_range_Ia/1 -> jmp_cnt18_ph/7(in_range_Ia), Ia_diff_calc/8(in_range_I)
  9/1 -> Ic_calc/5(K_CT), Ia_calc/5(K_CT), Ib_calc/5(K_CT)
  6/1 -> Ic_calc/8(Fi_CT), Ia_calc/8(Fi_CT), Ib_calc/8(Fi_CT)
  Fi_T/1 -> Ic_calc/9(Fi_T), Ia_calc/9(Fi_T), Ib_calc/9(Fi_T)
  I0_comp/1 -> Ic_calc/7(I0_comp), Ia_calc/7(I0_comp), Ib_calc/7(I0_comp)
  K_T/1 -> Ic_calc/6(K_T), Ib_calc/6(K_T), Ia_calc/6(K_T)

== system mylib/278_dzt_v1/diff_trans_calc_H1 ==
  Ia_re_diff_in : Inport
  Ia_im_diff_in : Inport  Port=2
  Ia_re_max_in : Inport  Port=3
  Ia_im_max_in : Inport  Port=4
  Ib_re_diff_in : Inport  Port=5
  Ib_im_diff_in : Inport  Port=6
  Ib_re_max_in : Inport  Port=7
  Ib_im_max_in : Inport  Port=8
  Ic_re_diff_in : Inport  Port=9
  Ic_im_diff_in : Inport  Port=10
  Ic_re_max_in : Inport  Port=11
  Ic_im_max_in : Inport  Port=12
  Ia_zero_in : Inport  Port=13
  Ib_zero_in : Inport  Port=14
  Ic_zero_in : Inport  Port=15
  I_all_zero_in : Inport  Port=16
  Ia_re : Inport  Port=17
  Ia_im : Inport  Port=18
  Ib_re : Inport  Port=19
  Ib_im : Inport  Port=20
  Ic_re : Inport  Port=21
  Ic_im : Inport  Port=22
  jmp_a : Inport  Port=23
  jmp_b : Inport  Port=24
  jmp_c : Inport  Port=25
  in_range_Ia : Inport  Port=26
  in_range_Ib : Inport  Port=27
  in_range_Ic : Inport  Port=28
  K_T : Inport  Port=29
  I0_comp : Inport  Port=30
  Fi_T : Inport  Port=31
  1 : Constant  Value=0
  2 : Constant
  6 : Constant  Value=0
  9 : Constant
  Ia_calc : Subsystem
  Ia_diff_calc : Subsystem
  Ib_calc : Subsystem
  Ib_diff_calc : Subsystem
  Ic_calc : Subsystem
  Ic_diff_calc : Subsystem
  jmp_cnt18_ph : Subsystem
  simpcomp : Subsystem
  Ia_re_diff : Outport
  Ia_im_diff : Outport  Port=2
  Ia_re_max : Outport  Port=3
  Ia_im_max : Outport  Port=4
  Ib_re_diff : Outport  Port=5
  Ib_im_diff : Outport  Port=6
  Ib_re_max : Outport  Port=7
  Ib_im_max : Outport  Port=8
  Ic_re_diff : Outport  Port=9
  Ic_im_diff : Outport  Port=10
  Ic_re_max : Outport  Port=11
  Ic_im_max : Outport  Port=12
  Ia_zero : Outport  Port=13
  Ib_zero : Outport  Port=14
  Ic_zero : Outport  Port=15
  I_all_zero : Outport  Port=16
  wires:
  Ia_re/1 -> simpcomp/1(FAre), Ia_calc/1(I_re_in)
  I_all_zero_in/1 -> jmp_cnt18_ph/6(Iall_zero_in)
  Ic_zero_in/1 -> jmp_cnt18_ph/5(Ic_zero_in)
  Ib_zero_in/1 -> jmp_cnt18_ph/4(Ib_zero_in)
  Ia_zero_in/1 -> jmp_cnt18_ph/3(Ia_zero_in)
  Ic_im_max_in/1 -> Ic_diff_calc/7(I_im_max_in)
  Ic_re_max_in/1 -> Ic_diff_calc/6(I_re_max_in)
  Ic_im_diff_in/1 -> Ic_diff_calc/2(I_im_1)
  Ic_re_diff_in/1 -> Ic_diff_calc/1(I_re_1)
  Ib_im_max_in/1 -> Ib_diff_calc/7(I_im_max_in)
  Ib_re_max_in/1 -> Ib_diff_calc/6(I_re_max_in)
  Ib_im_diff_in/1 -> Ib_diff_calc/2(I_im_1)
  Ib_re_diff_in/1 -> Ib_diff_calc/1(I_re_1)
  Ia_im_max_in/1 -> Ia_diff_calc/7(I_im_max_in)
  Ia_re_max_in/1 -> Ia_diff_calc/6(I_re_max_in)
  Ia_im_diff_in/1 -> Ia_diff_calc/2(I_im_1)
  Ia_re_diff_in/1 -> Ia_diff_calc/1(I_re_1)
  2/1 -> Ia_diff_calc/5(fix), Ib_diff_calc/5(fix), jmp_cnt18_ph/13(fix), Ic_diff_calc/5(fix)
  1/1 -> jmp_cnt18_ph/2(cnt_jmp_in), jmp_cnt18_ph/1(cnt_jmp0_in)
  Ia_calc/1(I_re) -> Ia_diff_calc/3(I_re_2)
  Ia_calc/2(I_im) -> Ia_diff_calc/4(I_im_2)
  Ib_calc/1(I_re) -> Ib_diff_calc/3(I_re_2)
  Ib_calc/2(I_im) -> Ib_diff_calc/4(I_im_2)
  Ic_calc/1(I_re) -> Ic_diff_calc/3(I_re_2)
  Ic_calc/2(I_im) -> Ic_diff_calc/4(I_im_2)
  Ia_diff_calc/1(I_re_diff) -> Ia_re_diff/1
  Ia_diff_calc/2(I_im_diff1) -> Ia_im_diff/1
  Ia_diff_calc/3(I_re_max) -> Ia_re_max/1
  Ia_diff_calc/4(I_im_max) -> Ia_im_max/1
  Ib_diff_calc/4(I_im_max) -> Ib_im_max/1
  Ib_diff_calc/3(I_re_max) -> Ib_re_max/1
  Ib_diff_calc/2(I_im_diff1) -> Ib_im_diff/1
  Ib_diff_calc/1(I_re_diff) -> Ib_re_diff/1
  Ic_diff_calc/4(I_im_max) -> Ic_im_max/1
  Ic_diff_calc/3(I_re_max) -> Ic_re_max/1
  Ic_diff_calc/2(I_im_diff1) -> Ic_im_diff/1
  Ic_diff_calc/1(I_re_diff) -> Ic_re_diff/1
  jmp_cnt18_ph/6(Iall_zero) -> I_all_zero/1
  jmp_cnt18_ph/5(Ic_zero) -> Ic_zero/1
  jmp_cnt18_ph/4(Ib_zero) -> Ib_zero/1
  jmp_cnt18_ph/3(Ia_zero) -> Ia_zero/1
  Ia_im/1 -> simpcomp/2(FAim), Ia_calc/2(I_im_in)
  Ib_re/1 -> simpcomp/3(FBre), Ib_calc/1(I_re_in)
  Ib_im/1 -> simpcomp/4(FBim), Ib_calc/2(I_im_in)
  Ic_re/1 -> simpcomp/5(FCre), Ic_calc/1(I_re_in)
  Ic_im/1 -> simpcomp/6(FCim), Ic_calc/2(I_im_in)
  jmp_a/1 -> jmp_cnt18_ph/10(jmp_Ia)
  jmp_b/1 -> jmp_cnt18_ph/11(jmp_Ib)
  jmp_c/1 -> jmp_cnt18_ph/12(jmp_Ic)
  in_range_Ib/1 -> jmp_cnt18_ph/8(in_range_Ib), Ib_diff_calc/8(in_range_I)
  in_range_Ic/1 -> Ic_diff_calc/8(in_range_I), jmp_cnt18_ph/9(in_range_Ic)
  simpcomp/2(F0im) -> Ib_calc/4(I30_im), Ia_calc/4(I30_im), Ic_calc/4(I30_im)
  simpcomp/1(F0re) -> Ia_calc/3(I30_re), Ib_calc/3(I30_re), Ic_calc/3(I30_re)
  in_range_Ia/1 -> jmp_cnt18_ph/7(in_range_Ia), Ia_diff_calc/8(in_range_I)
  9/1 -> Ic_calc/5(K_CT), Ia_calc/5(K_CT), Ib_calc/5(K_CT)
  6/1 -> Ic_calc/8(Fi_CT), Ia_calc/8(Fi_CT), Ib_calc/8(Fi_CT)
  Fi_T/1 -> Ic_calc/9(Fi_T), Ia_calc/9(Fi_T), Ib_calc/9(Fi_T)
  I0_comp/1 -> Ic_calc/7(I0_comp), Ia_calc/7(I0_comp), Ib_calc/7(I0_comp)
  K_T/1 -> Ic_calc/6(K_T), Ib_calc/6(K_T), Ia_calc/6(K_T)

== system mylib/278_dzt_v1/diff_trans_calc_H2 ==
  Ia_re_diff_in : Inport
  Ia_im_diff_in : Inport  Port=2
  Ia_re_max_in : Inport  Port=3
  Ia_im_max_in : Inport  Port=4
  Ib_re_diff_in : Inport  Port=5
  Ib_im_diff_in : Inport  Port=6
  Ib_re_max_in : Inport  Port=7
  Ib_im_max_in : Inport  Port=8
  Ic_re_diff_in : Inport  Port=9
  Ic_im_diff_in : Inport  Port=10
  Ic_re_max_in : Inport  Port=11
  Ic_im_max_in : Inport  Port=12
  Ia_zero_in : Inport  Port=13
  Ib_zero_in : Inport  Port=14
  Ic_zero_in : Inport  Port=15
  I_all_zero_in : Inport  Port=16
  Ia_re : Inport  Port=17
  Ia_im : Inport  Port=18
  Ib_re : Inport  Port=19
  Ib_im : Inport  Port=20
  Ic_re : Inport  Port=21
  Ic_im : Inport  Port=22
  jmp_a : Inport  Port=23
  jmp_b : Inport  Port=24
  jmp_c : Inport  Port=25
  in_range_Ia : Inport  Port=26
  in_range_Ib : Inport  Port=27
  in_range_Ic : Inport  Port=28
  K_T : Inport  Port=29
  I0_comp : Inport  Port=30
  Fi_T : Inport  Port=31
  1 : Constant  Value=0
  2 : Constant
  6 : Constant  Value=0
  9 : Constant
  Ia_calc : Subsystem
  Ia_diff_calc : Subsystem
  Ib_calc : Subsystem
  Ib_diff_calc : Subsystem
  Ic_calc : Subsystem
  Ic_diff_calc : Subsystem
  jmp_cnt18_ph : Subsystem
  simpcomp : Subsystem
  Ia_re_diff : Outport
  Ia_im_diff : Outport  Port=2
  Ia_re_max : Outport  Port=3
  Ia_im_max : Outport  Port=4
  Ib_re_diff : Outport  Port=5
  Ib_im_diff : Outport  Port=6
  Ib_re_max : Outport  Port=7
  Ib_im_max : Outport  Port=8
  Ic_re_diff : Outport  Port=9
  Ic_im_diff : Outport  Port=10
  Ic_re_max : Outport  Port=11
  Ic_im_max : Outport  Port=12
  Ia_zero : Outport  Port=13
  Ib_zero : Outport  Port=14
  Ic_zero : Outport  Port=15
  I_all_zero : Outport  Port=16
  wires:
  Ia_re/1 -> simpcomp/1(FAre), Ia_calc/1(I_re_in)
  I_all_zero_in/1 -> jmp_cnt18_ph/6(Iall_zero_in)
  Ic_zero_in/1 -> jmp_cnt18_ph/5(Ic_zero_in)
  Ib_zero_in/1 -> jmp_cnt18_ph/4(Ib_zero_in)
  Ia_zero_in/1 -> jmp_cnt18_ph/3(Ia_zero_in)
  Ic_im_max_in/1 -> Ic_diff_calc/7(I_im_max_in)
  Ic_re_max_in/1 -> Ic_diff_calc/6(I_re_max_in)
  Ic_im_diff_in/1 -> Ic_diff_calc/2(I_im_1)
  Ic_re_diff_in/1 -> Ic_diff_calc/1(I_re_1)
  Ib_im_max_in/1 -> Ib_diff_calc/7(I_im_max_in)
  Ib_re_max_in/1 -> Ib_diff_calc/6(I_re_max_in)
  Ib_im_diff_in/1 -> Ib_diff_calc/2(I_im_1)
  Ib_re_diff_in/1 -> Ib_diff_calc/1(I_re_1)
  Ia_im_max_in/1 -> Ia_diff_calc/7(I_im_max_in)
  Ia_re_max_in/1 -> Ia_diff_calc/6(I_re_max_in)
  Ia_im_diff_in/1 -> Ia_diff_calc/2(I_im_1)
  Ia_re_diff_in/1 -> Ia_diff_calc/1(I_re_1)
  2/1 -> Ia_diff_calc/5(fix), Ib_diff_calc/5(fix), jmp_cnt18_ph/13(fix), Ic_diff_calc/5(fix)
  1/1 -> jmp_cnt18_ph/2(cnt_jmp_in), jmp_cnt18_ph/1(cnt_jmp0_in)
  Ia_calc/1(I_re) -> Ia_diff_calc/3(I_re_2)
  Ia_calc/2(I_im) -> Ia_diff_calc/4(I_im_2)
  Ib_calc/1(I_re) -> Ib_diff_calc/3(I_re_2)
  Ib_calc/2(I_im) -> Ib_diff_calc/4(I_im_2)
  Ic_calc/1(I_re) -> Ic_diff_calc/3(I_re_2)
  Ic_calc/2(I_im) -> Ic_diff_calc/4(I_im_2)
  Ia_diff_calc/1(I_re_diff) -> Ia_re_diff/1
  Ia_diff_calc/2(I_im_diff1) -> Ia_im_diff/1
  Ia_diff_calc/3(I_re_max) -> Ia_re_max/1
  Ia_diff_calc/4(I_im_max) -> Ia_im_max/1
  Ib_diff_calc/4(I_im_max) -> Ib_im_max/1
  Ib_diff_calc/3(I_re_max) -> Ib_re_max/1
  Ib_diff_calc/2(I_im_diff1) -> Ib_im_diff/1
  Ib_diff_calc/1(I_re_diff) -> Ib_re_diff/1
  Ic_diff_calc/4(I_im_max) -> Ic_im_max/1
  Ic_diff_calc/3(I_re_max) -> Ic_re_max/1
  Ic_diff_calc/2(I_im_diff1) -> Ic_im_diff/1
  Ic_diff_calc/1(I_re_diff) -> Ic_re_diff/1
  jmp_cnt18_ph/6(Iall_zero) -> I_all_zero/1
  jmp_cnt18_ph/5(Ic_zero) -> Ic_zero/1
  jmp_cnt18_ph/4(Ib_zero) -> Ib_zero/1
  jmp_cnt18_ph/3(Ia_zero) -> Ia_zero/1
  Ia_im/1 -> simpcomp/2(FAim), Ia_calc/2(I_im_in)
  Ib_re/1 -> simpcomp/3(FBre), Ib_calc/1(I_re_in)
  Ib_im/1 -> simpcomp/4(FBim), Ib_calc/2(I_im_in)
  Ic_re/1 -> simpcomp/5(FCre), Ic_calc/1(I_re_in)
  Ic_im/1 -> simpcomp/6(FCim), Ic_calc/2(I_im_in)
  jmp_a/1 -> jmp_cnt18_ph/10(jmp_Ia)
  jmp_b/1 -> jmp_cnt18_ph/11(jmp_Ib)
  jmp_c/1 -> jmp_cnt18_ph/12(jmp_Ic)
  in_range_Ib/1 -> jmp_cnt18_ph/8(in_range_Ib), Ib_diff_calc/8(in_range_I)
  in_range_Ic/1 -> Ic_diff_calc/8(in_range_I), jmp_cnt18_ph/9(in_range_Ic)
  simpcomp/2(F0im) -> Ib_calc/4(I30_im), Ia_calc/4(I30_im), Ic_calc/4(I30_im)
  simpcomp/1(F0re) -> Ia_calc/3(I30_re), Ib_calc/3(I30_re), Ic_calc/3(I30_re)
  in_range_Ia/1 -> jmp_cnt18_ph/7(in_range_Ia), Ia_diff_calc/8(in_range_I)
  9/1 -> Ic_calc/5(K_CT), Ia_calc/5(K_CT), Ib_calc/5(K_CT)
  6/1 -> Ic_calc/8(Fi_CT), Ia_calc/8(Fi_CT), Ib_calc/8(Fi_CT)
  Fi_T/1 -> Ic_calc/9(Fi_T), Ia_calc/9(Fi_T), Ib_calc/9(Fi_T)
  I0_comp/1 -> Ic_calc/7(I0_comp), Ia_calc/7(I0_comp), Ib_calc/7(I0_comp)
  K_T/1 -> Ic_calc/6(K_T), Ib_calc/6(K_T), Ia_calc/6(K_T)

== system mylib/278_dzt_v1/i_ctl18_ph ==
  cnt_jmp0 : Inport
  cnt_jmp : Inport  Port=2
  Ia_diff : Inport  Port=3
  Ib_diff : Inport  Port=4
  Ic_diff : Inport  Port=5
  Ia_zero : Inport  Port=6
  Ib_zero : Inport  Port=7
  Ic_zero : Inport  Port=8
  I_ctl_led : Inport  Port=9
  "I_unb " : Inport  Port=10
  1 : RelationalOperator  Operator=>  OutDataTypeStr=boolean  RndMeth=Simplest
  {4..6,10,12} (5 alike) : Logic  AllPortsSameDT=off  OutDataTypeStr=boolean
  11 : Logic  Operator=OR  Inputs=3  AllPortsSameDT=off  OutDataTypeStr=boolean
  13 : Logic  Operator=NOT  AllPortsSameDT=off  OutDataTypeStr=boolean
  14 : Logic  Operator=OR  AllPortsSameDT=off  OutDataTypeStr=boolean
  2 : RelationalOperator  Operator=>  OutDataTypeStr=boolean  RndMeth=Simplest
  3 : RelationalOperator  Operator=>  OutDataTypeStr=boolean  RndMeth=Simplest
  7 : Constant
  8 : RelationalOperator  Operator===  OutDataTypeStr=boolean  RndMeth=Simplest
  9 : RelationalOperator  Operator===  OutDataTypeStr=boolean  RndMeth=Simplest
  R_TRIG : $bdroot/R_TRIG  SystemSampleTime=-1  Latency=0  AutoFrameSizeCalculation=off
  T1 : powerlib_meascontrol/Logic/On Delay  DelayType=Off delay  delay=T_I_ctl  ic=1  Ts=0
  T2 : powerlib_meascontrol/Logic/On Delay  DelayType=Off delay  delay=T_I_ctl  ic=1  Ts=0
  T3 : powerlib_meascontrol/Logic/On Delay  DelayType=Off delay  delay=T_I_ctl  ic=1  Ts=0
  avar : Outport
  block : Outport  Port=2
  led : Outport  Port=3
  jmp_unb : Outport  Port=4
  I_unb : Outport  Port=5
  Ia_unb : Outport  Port=6
  Ib_unb : Outport  Port=7
  Ic_unb : Outport  Port=8
  wires:
  12/1 -> block/1
  R_TRIG/1 -> avar/1
  I_ctl_led/1 -> 13/1
  14/1 -> 12/1, R_TRIG/1, led/1
  13/1 -> 12/2
  10/1 -> jmp_unb/1, 14/1
  11/1 -> I_unb/1, 14/2
  T1/1 -> 11/1, Ia_unb/1
  T2/1 -> 11/2, Ib_unb/1
  T3/1 -> 11/3, Ic_unb/1
  5/1 -> T2/1
  6/1 -> T3/1
  4/1 -> T1/1
  9/1 -> 10/2
  8/1 -> 10/1
  cnt_jmp/1 -> 9/1
  cnt_jmp0/1 -> 8/1
  7/1 -> 8/2, 9/2
  Ic_zero/1 -> 6/2
  Ib_zero/1 -> 5/2
  Ia_zero/1 -> 4/2
  "I_unb "/1 -> 1/2, 2/2, 3/2
  Ic_diff/1 -> 3/1
  Ib_diff/1 -> 2/1
  3/1 -> 6/1
  2/1 -> 5/1
  1/1 -> 4/1
  Ia_diff/1 -> 1/1

== system mylib/278_dzt_v1/out1 ==
  in : Inport
  1 : Logic  Operator=OR  AllPortsSameDT=off  OutDataTypeStr=boolean
  2 : powerlib_meascontrol/Logic/Monostable  EdgeDetect=Rising  PulseDuration=T_out  ic=0  Ts=0
      settings: SourceProductBaseCode=PS
  R_TRIG : $bdroot/R_TRIG  SystemSampleTime=-1  Latency=0  AutoFrameSizeCalculation=off
  out : Outport
  wires:
  2/1 -> 1/2
  1/1 -> out/1
  R_TRIG/1 -> 1/1
  in/1 -> R_TRIG/1, 2/1

== system mylib/278_dzt_v1/out2 ==
  in : Inport
  1 : Logic  Operator=OR  AllPortsSameDT=off  OutDataTypeStr=boolean
  2 : powerlib_meascontrol/Logic/Monostable  EdgeDetect=Rising  PulseDuration=T_out  ic=0  Ts=0
      settings: SourceProductBaseCode=PS
  R_TRIG : $bdroot/R_TRIG  SystemSampleTime=-1  Latency=0  AutoFrameSizeCalculation=off
  out : Outport
  wires:
  2/1 -> 1/2
  1/1 -> out/1
  R_TRIG/1 -> 1/1
  in/1 -> R_TRIG/1, 2/1

== system mylib/278_dzt_v1/out3 ==
  in : Inport
  1 : Logic  Operator=OR  AllPortsSameDT=off  OutDataTypeStr=boolean
  2 : powerlib_meascontrol/Logic/Monostable  EdgeDetect=Rising  PulseDuration=T_out  ic=0  Ts=0
      settings: SourceProductBaseCode=PS
  R_TRIG : $bdroot/R_TRIG  SystemSampleTime=-1  Latency=0  AutoFrameSizeCalculation=off
  out : Outport
  wires:
  2/1 -> 1/2
  1/1 -> out/1
  R_TRIG/1 -> 1/1
  in/1 -> R_TRIG/1, 2/1

== system mylib/339_i_recalc_ph_v1/I0_1 ==
  Re : Inport
  Im : Inport  Port=2
  1 : Product  Inputs=**
  2 : Sum
  3 : Product  Inputs=**
  4 : Sqrt  SaturateOnIntegerOverflow=on
  Module : Outport
  wires:
  3/1 -> 2/2
  1/1 -> 2/1
  Im/1 -> 3/1, 3/2
  4/1 -> Module/1
  2/1 -> 4/1
  Re/1 -> 1/2, 1/1

== system mylib/339_i_recalc_ph_v1/I0_2 ==
  Re : Inport
  Im : Inport  Port=2
  1 : Product  Inputs=**
  2 : Sum
  3 : Product  Inputs=**
  4 : Sqrt  SaturateOnIntegerOverflow=on
  Module : Outport
  wires:
  3/1 -> 2/2
  1/1 -> 2/1
  Im/1 -> 3/1, 3/2
  4/1 -> Module/1
  2/1 -> 4/1
  Re/1 -> 1/2, 1/1

== system mylib/339_i_recalc_ph_v1/Ia1 ==
  Re : Inport
  Im : Inport  Port=2
  1 : Product  Inputs=**
  2 : Sum
  3 : Product  Inputs=**
  4 : Sqrt  SaturateOnIntegerOverflow=on
  Module : Outport
  wires:
  3/1 -> 2/2
  1/1 -> 2/1
  Im/1 -> 3/1, 3/2
  4/1 -> Module/1
  2/1 -> 4/1
  Re/1 -> 1/2, 1/1

== system mylib/339_i_recalc_ph_v1/Ia2 ==
  Re : Inport
  Im : Inport  Port=2
  1 : Product  Inputs=**
  2 : Sum
  3 : Product  Inputs=**
  4 : Sqrt  SaturateOnIntegerOverflow=on
  Module : Outport
  wires:
  3/1 -> 2/2
  1/1 -> 2/1
  Im/1 -> 3/1, 3/2
  4/1 -> Module/1
  2/1 -> 4/1
  Re/1 -> 1/2, 1/1

== system mylib/339_i_recalc_ph_v1/Ib1 ==
  Re : Inport
  Im : Inport  Port=2
  1 : Product  Inputs=**
  2 : Sum
  3 : Product  Inputs=**
  4 : Sqrt  SaturateOnIntegerOverflow=on
  Module : Outport
  wires:
  3/1 -> 2/2
  1/1 -> 2/1
  Im/1 -> 3/1, 3/2
  4/1 -> Module/1
  2/1 -> 4/1
  Re/1 -> 1/2, 1/1

== system mylib/339_i_recalc_ph_v1/Ib2 ==
  Re : Inport
  Im : Inport  Port=2
  1 : Product  Inputs=**
  2 : Sum
  3 : Product  Inputs=**
  4 : Sqrt  SaturateOnIntegerOverflow=on
  Module : Outport
  wires:
  3/1 -> 2/2
  1/1 -> 2/1
  Im/1 -> 3/1, 3/2
  4/1 -> Module/1
  2/1 -> 4/1
  Re/1 -> 1/2, 1/1

== system mylib/339_i_recalc_ph_v1/Ic1 ==
  Re : Inport
  Im : Inport  Port=2
  1 : Product  Inputs=**
  2 : Sum
  3 : Product  Inputs=**
  4 : Sqrt  SaturateOnIntegerOverflow=on
  Module : Outport
  wires:
  3/1 -> 2/2
  1/1 -> 2/1
  Im/1 -> 3/1, 3/2
  4/1 -> Module/1
  2/1 -> 4/1
  Re/1 -> 1/2, 1/1

== system mylib/339_i_recalc_ph_v1/Ic2 ==
  Re : Inport
  Im : Inport  Port=2
  1 : Product  Inputs=**
  2 : Sum
  3 : Product  Inputs=**
  4 : Sqrt  SaturateOnIntegerOverflow=on
  Module : Outport
  wires:
  3/1 -> 2/2
  1/1 -> 2/1
  Im/1 -> 3/1, 3/2
  4/1 -> Module/1
  2/1 -> 4/1
  Re/1 -> 1/2, 1/1
